simulink model "accsim"  (Simulink 7.7)
settings: Solver=ode45  StartTime=0.0  StopTime=25.0  RelTol=1e-3
values from neighbouring files (symbols this model uses):
  kd = -c0+m0*(p+2*zeta*wn)    (= 4210.3)    [acc.m]
  ki = m0*wn^2*p    (= 556.25)    [acc.m]
  kp = m0*(2*zeta*wn*p+wn^2)    (= 2558.75)    [acc.m]
  r_desired = 30    [acc.m]
  tau = .01    (= 0.01)    [acc.m]
  v0 = reftraj.vp(1)    [acc.m]
libraries: simulink_need_slupdate x1, RCTblocks x1
settings Model: Creator=guiness  LastModifiedBy=pseiler  ExtModeAutoUpdateStatusClock=off
settings OptimizationCC: BooleanDataType=off
settings DebuggingCC: SaveWithParameterizedLinksMsg=none  SignalResolutionControl=TryResolveAllWithWarning  SolverPrmCheckMsg=none  MultiTaskDSMMsg=warning  MultiTaskCondExecSysMsg=none  FcnCallInpInsideContextMsg=Enable All  StrictBusMsg=None
settings HardwareCC: TargetUnknown=on
settings RTWCC: IncludeERTFirstTime=on

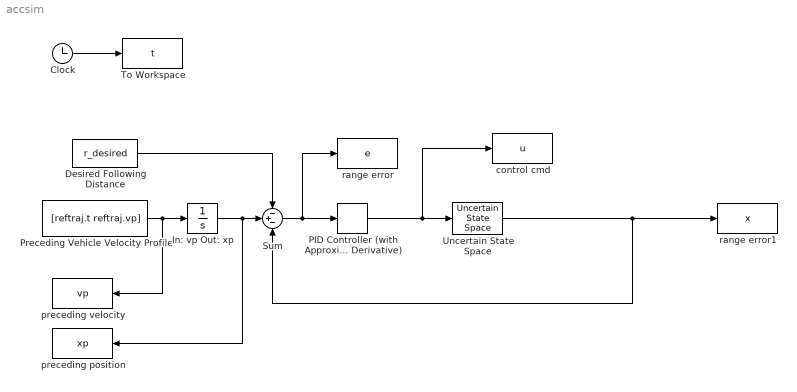
== system accsim ==
  Clock : Clock
      settings: Decimation=10
  Desired Following Distance : Constant  Value=r_desired
  In: vp Out: xp : Integrator  InitialCondition=r_desired
  PID Controller (with Approximate Derivative) : simulink_need_slupdate/PID Controller (with Approximate Derivative)  SystemSampleTime=-1  P=kp  I=ki  D=kd  N=1/tau
  Preceding Vehicle Velocity Profile : FromWorkspace  VariableName=[reftraj.t reftraj.vp]  SampleTime=0.01
  Sum : Sum  Inputs=-+-  SaturateOnIntegerOverflow=on  InputSameDT=on  OutDataTypeStr=Inherit: Same as first input
  To Workspace : ToWorkspace  VariableName=t  SampleTime=-1  SaveFormat=Array
  Uncertain State Space : RCTblocks/Uncertain State Space  Tag=USS  SystemSampleTime=-1  USystem=P  UValue=V  X0=[0 v0 0]  uX0=[]
  control cmd : ToWorkspace  VariableName=u  SampleTime=-1  SaveFormat=Array
  preceding position : ToWorkspace  VariableName=xp  SampleTime=-1  SaveFormat=Array
  preceding velocity : ToWorkspace  VariableName=vp  SaveFormat=Array
  range error : ToWorkspace  VariableName=e  SampleTime=-1  SaveFormat=Array
  range error1 : ToWorkspace  VariableName=x  SampleTime=-1  SaveFormat=Array
  wires:
  Clock/1 -> To Workspace/1
  Preceding Vehicle Velocity Profile/1 -> In: vp Out: xp/1, preceding velocity/1
  PID Controller (with Approximate Derivative)/1 -> Uncertain State Space/1, control cmd/1
  In: vp Out: xp/1 -> Sum/2, preceding position/1
  Desired Following Distance/1 -> Sum/1
  Uncertain State Space/1 -> Sum/3, range error1/1
  Sum/1 -> PID Controller (with Approximate Derivative)/1, range error/1
